simulink subsystem "joyToPWM"  (R2025b)
settings: Solver=VariableStepAuto  StartTime=0.0  StopTime=10.0  RelTol=1e-3
undefined symbols (not defined in the file): masks, max_thruster_force
settings Model: Creator=kjhaydon  LastModifiedBy=kjhaydon

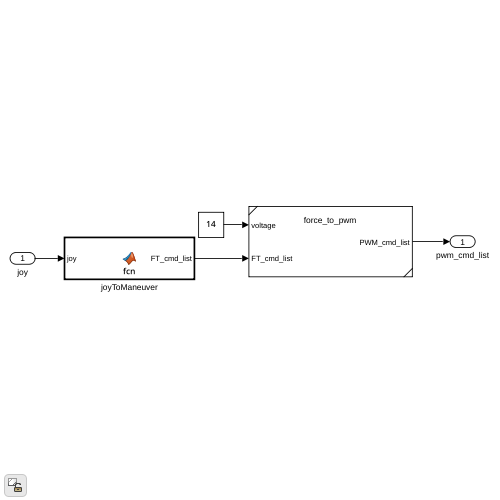
[thumbnail: Simulink's stored preview of the top-level diagram]
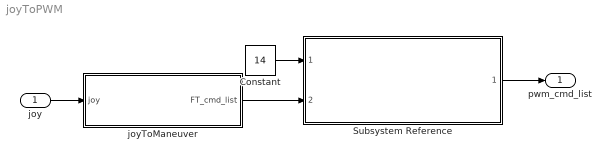
== system joyToPWM ==
  joy : Inport
  Constant : Constant  Value=14
  Subsystem Reference : Subsystem  ReferencedSubsystem=force_to_pwm
  joyToManeuver : MATLAB Function  TreatAsAtomicUnit=on
  pwm_cmd_list : Outport
  wires:
  joy/1 -> joyToManeuver/1(joy)
  joyToManeuver/1(FT_cmd_list) -> Subsystem Reference/2
  Subsystem Reference/1 -> pwm_cmd_list/1
  Constant/1 -> Subsystem Reference/1

== matlab function joyToPWM/joyToManeuver ==
  data: joy input; FT_cmd_list output; masks parameter; max_thruster_force parameter
function FT_cmd_list = fcn(joy,masks, max_thruster_force)

FT_cmd_list = joyToManeuver(joy,masks,max_thruster_force);
